simulink model "dqn_C_PQ_HVsMC"  (R2024a)
settings: Solver=FixedStepDiscrete  StartTime=0.0  StopTime=10  FixedStep=Ts_Power  RelTol=1e-3
PreLoadFcn:
  | % HVDCMMCInterconnectionParam
StartFcn:
  | tic
StopFcn:
  | toc
values from neighbouring files (symbols this model uses):
  C_PM = 1.758e-3    (= 0.001758)    [dqnMMCsingle.m]
  Fnom = 50    [dqnMMCsingle.m]
  HRM = 1    [dqnMMCsingle.m]
  Ki_Ireg = 6    [dqnMMCsingle.m]
  Ki_Qreg = 1.0    (= 1)    [dqnMMCsingle.m]
  Kp_Ireg = 0.6    [dqnMMCsingle.m]
  Kp_Qreg = 0.5/3    (= 0.166666666667)    [dqnMMCsingle.m]
  Larm = Larm_pu*(Zb_ac/(2*pi*Fnom))    [dqnMMCsingle.m]
  Larm_pu = 0.15    [dqnMMCsingle.m]
  Lff = Larm_pu/2    (= 0.075)    [dqnMMCsingle.m]
  Limits_Ireg = [ 2.0  -2.0]    [dqnMMCsingle.m]
  Limits_Qreg = [ 0.25, -0.25 ]    [dqnMMCsingle.m]
  Limits_VDCreg = [ 2.0  -2.0]    [dqnMMCsingle.m]
  Lxfo = 0.12    [dqnMMCsingle.m]
  N = 1    [dqnMMCsingle.m]
  Nb_PM = 36    [dqnMMCsingle.m]
  Pnom = 1000e6    (= 1000000000)    [dqnMMCsingle.m]
  R_startup = 400    [dqnMMCsingle.m]
  Rarm = Rarm_pu*Zb_ac    [dqnMMCsingle.m]
  Rff = Rarm_pu/2    (= 0.00075)    [dqnMMCsingle.m]
  Rxfo = 0.003    [dqnMMCsingle.m]
  Slope_Qref = 0.5    [dqnMMCsingle.m]
  Slope_Vdc_ref = Vnom_dc/5    (= 128000)    [dqnMMCsingle.m]
  Tfault = 9999    [dqnMMCsingle.m]
  Ts = Ts_Control    (= 4e-05)    [dqnMMCsingle.m]
  Ts_Control = 40e-6    (= 4e-05)    [dqnMMCsingle.m]
  Ts_dqn = 2e-5    (= 2e-05)    [dqnMMCsingle.m]
  Ts_Power = 20e-6    (= 2e-05)    [dqnMMCsingle.m]
  Vnom_dc = 640e3    (= 640000)    [dqnMMCsingle.m]
  Vnom_prim = 400e3    (= 400000)    [dqnMMCsingle.m]
  Vnom_sec = 333e3    (= 333000)    [dqnMMCsingle.m]
  Ws = 2*pi*50    (= 314.159265359)    [dqnMMCsingle.m]
undefined symbols (not defined in the file or in its folder): DiscIntNeverNeededParam, Discrete, DQN_Lib, gcbh, Int_DQNc_Mat, Mult_DQNc_Mat, Pcc, S, sps, sps_rtmsupport, spsMeanValueVariableFrequencyModel, spsPLL3phModel, SY3
libraries: simulink x18, spsControlledVoltageSourceLib x15, spsVoltageMeasurementLib x9, powerlib_extras x6, spsSecondOrderFilterLib x6, spsCurrentMeasurementLib x6, spsIdealSwitchLib x6, spsMeanLib x4, spsdq0toabcLib x4, spsMeanVariableFrequencyLib x4, spsabctodq0Lib x4, spsThreePhaseSeriesRLCBranchLib x4
(part 3 of 6)

== system dqn_C_PQ_HVsMC/Controllers1/Current Regulator (Ireg)/PI regulator with anti-windup Q ==
  note: Anti-windup mechanism: Method of conditionnal integration
      |
      | The integration is suspended if saturation occurs and the
      | control error is of the same sign as the control signal.
      |
      | [1] L.Rundqwist, "Anti-Reset Windup for PID Controllers," Ph.D. Thesis TRFT-1033,
      | Departement of Automatic Control, Lund Institute of Technology, Lund, Sweeden, 1991.
  Error : Inport  SampleTime=Ts
  Compare To Zero : simulink/Logic and Bit Operations/Compare To Zero  relop=>  OutDataTypeStr=uint8  ZeroCross=off
  Compare To Zero1 : simulink/Logic and Bit Operations/Compare To Zero  relop=<  OutDataTypeStr=uint8  ZeroCross=off
  Constant : Constant  Value=0
  Constant1 : Constant  Value=UpperLimit
  Constant3 : Constant  Value=LowerLimit
  Discrete-Time Integrator : DiscreteIntegrator  IntegratorMethod=Integration: Trapezoidal  InitialCondition=Init  SampleTime=Ts  LimitOutput=on  UpperSaturationLimit=UpperLimit  LowerSaturationLimit=LowerLimit  ShowStatePort=on  ICPrevOutput=DiscIntNeverNeededParam  ICPrevScaledInput=DiscIntNeverNeededParam
  Kp4 : Gain  Gain=Kp  SaturateOnIntegerOverflow=on  SampleTime=Ts  OutDataTypeStr=Inherit: Same as input  ParamDataTypeStr=Inherit: Same as input
  Kp5 : Gain  Gain=Ki  SaturateOnIntegerOverflow=on  SampleTime=Ts  OutDataTypeStr=Inherit: Same as input  ParamDataTypeStr=Inherit: Same as input
  Logical Operator : Logic  AllPortsSameDT=off  OutDataTypeStr=boolean
  Logical Operator1 : Logic  AllPortsSameDT=off  OutDataTypeStr=boolean
  Logical Operator2 : Logic  Operator=OR  AllPortsSameDT=off  OutDataTypeStr=boolean
  Relational Operator : RelationalOperator  OutDataTypeStr=boolean  InputSameDT=off
  Relational Operator1 : RelationalOperator  Operator=<=  OutDataTypeStr=boolean  InputSameDT=off
  Saturation2 : Saturate  UpperLimit=UpperLimit  LowerLimit=LowerLimit  SampleTime=Ts
  Sum1 : Sum  InputSameDT=on  SaturateOnIntegerOverflow=on  SampleTime=Ts  OutDataTypeStr=Inherit: Same as first input
  Sum6 : Sum  InputSameDT=on  SaturateOnIntegerOverflow=on  SampleTime=Ts  OutDataTypeStr=Inherit: Same as first input
  Switch : Switch  Criteria=u2 > Threshold  SaturateOnIntegerOverflow=off  InputSameDT=off
  Zero-Order Hold : ZeroOrderHold  SampleTime=Ts
  Out : Outport  SampleTime=Ts  InitialOutput=0
  wires:
  Kp5/1 -> Switch/3
  Switch/1 -> Discrete-Time Integrator/1
  Saturation2/1 -> Out/1
  Discrete-Time Integrator/1 -> Sum6/2
  Kp4/1 -> Zero-Order Hold/1
  Sum6/1 -> Saturation2/1
  Error/1 -> Kp5/1, Kp4/1, Compare To Zero/1, Compare To Zero1/1
  Compare To Zero1/1 -> Logical Operator1/2  "Error_is_negative"
  Logical Operator1/1 -> Logical Operator2/2
  Logical Operator/1 -> Logical Operator2/1
  Compare To Zero/1 -> Logical Operator/2  "Error_is_positive"
  Constant3/1 -> Relational Operator1/2
  Constant1/1 -> Relational Operator/2
  Relational Operator1/1 -> Logical Operator1/1  "LowerLimit_Is_Reached"
  Relational Operator/1 -> Logical Operator/1  "UpperLimit_is_Reached"
  Logical Operator2/1 -> Switch/2
  Sum1/1 -> Relational Operator/1, Relational Operator1/1
  Discrete-Time Integrator/State -> Sum1/1
  Zero-Order Hold/1 -> Sum6/1, Sum1/2
  Constant/1 -> Switch/1

== system dqn_C_PQ_HVsMC/DQsym/Circulating current suppression2/PI regulator with anti-windup D ==
  note: Anti-windup mechanism: Method of conditionnal integration
      |
      | The integration is suspended if saturation occurs and the
      | control error is of the same sign as the control signal.
      |
      | [1] L.Rundqwist, "Anti-Reset Windup for PID Controllers," Ph.D. Thesis TRFT-1033,
      | Departement of Automatic Control, Lund Institute of Technology, Lund, Sweeden, 1991.
  Error : Inport  SampleTime=Ts
  Compare To Zero : simulink/Logic and Bit Operations/Compare To Zero  relop=>  OutDataTypeStr=uint8  ZeroCross=off
  Compare To Zero1 : simulink/Logic and Bit Operations/Compare To Zero  relop=<  OutDataTypeStr=uint8  ZeroCross=off
  Constant : Constant  Value=0
  Constant1 : Constant  Value=UpperLimit
  Constant3 : Constant  Value=LowerLimit
  Discrete-Time Integrator : DiscreteIntegrator  IntegratorMethod=Integration: Trapezoidal  InitialCondition=Init  SampleTime=Ts  LimitOutput=on  UpperSaturationLimit=UpperLimit  LowerSaturationLimit=LowerLimit  ShowStatePort=on  ICPrevOutput=DiscIntNeverNeededParam  ICPrevScaledInput=DiscIntNeverNeededParam
  Kp4 : Gain  Gain=Kp  SaturateOnIntegerOverflow=on  SampleTime=Ts  OutDataTypeStr=Inherit: Same as input  ParamDataTypeStr=Inherit: Same as input
  Kp5 : Gain  Gain=Ki  SaturateOnIntegerOverflow=on  SampleTime=Ts  OutDataTypeStr=Inherit: Same as input  ParamDataTypeStr=Inherit: Same as input
  Logical Operator : Logic  AllPortsSameDT=off  OutDataTypeStr=boolean
  Logical Operator1 : Logic  AllPortsSameDT=off  OutDataTypeStr=boolean
  Logical Operator2 : Logic  Operator=OR  AllPortsSameDT=off  OutDataTypeStr=boolean
  Relational Operator : RelationalOperator  OutDataTypeStr=boolean  InputSameDT=off
  Relational Operator1 : RelationalOperator  Operator=<=  OutDataTypeStr=boolean  InputSameDT=off
  Saturation2 : Saturate  UpperLimit=UpperLimit  LowerLimit=LowerLimit  SampleTime=Ts
  Sum1 : Sum  InputSameDT=on  SaturateOnIntegerOverflow=on  SampleTime=Ts  OutDataTypeStr=Inherit: Same as first input
  Sum6 : Sum  InputSameDT=on  SaturateOnIntegerOverflow=on  SampleTime=Ts  OutDataTypeStr=Inherit: Same as first input
  Switch : Switch  Criteria=u2 > Threshold  SaturateOnIntegerOverflow=off  InputSameDT=off
  Zero-Order Hold : ZeroOrderHold  SampleTime=Ts
  Out : Outport  SampleTime=Ts  InitialOutput=0
  wires:
  Constant/1 -> Switch/1
  Zero-Order Hold/1 -> Sum1/2, Sum6/1
  Discrete-Time Integrator/State -> Sum1/1
  Sum1/1 -> Relational Operator1/1, Relational Operator/1
  Logical Operator2/1 -> Switch/2
  Relational Operator/1 -> Logical Operator/1  "UpperLimit_is_Reached"
  Relational Operator1/1 -> Logical Operator1/1  "LowerLimit_Is_Reached"
  Constant1/1 -> Relational Operator/2
  Constant3/1 -> Relational Operator1/2
  Compare To Zero/1 -> Logical Operator/2  "Error_is_positive"
  Logical Operator/1 -> Logical Operator2/1
  Logical Operator1/1 -> Logical Operator2/2
  Compare To Zero1/1 -> Logical Operator1/2  "Error_is_negative"
  Error/1 -> Compare To Zero1/1, Compare To Zero/1, Kp4/1, Kp5/1
  Sum6/1 -> Saturation2/1
  Kp4/1 -> Zero-Order Hold/1
  Discrete-Time Integrator/1 -> Sum6/2
  Saturation2/1 -> Out/1
  Switch/1 -> Discrete-Time Integrator/1
  Kp5/1 -> Switch/3

== system dqn_C_PQ_HVsMC/DQsym/Circulating current suppression2/PI regulator with anti-windup D1 ==
  note: Anti-windup mechanism: Method of conditionnal integration
      |
      | The integration is suspended if saturation occurs and the
      | control error is of the same sign as the control signal.
      |
      | [1] L.Rundqwist, "Anti-Reset Windup for PID Controllers," Ph.D. Thesis TRFT-1033,
      | Departement of Automatic Control, Lund Institute of Technology, Lund, Sweeden, 1991.
  Error : Inport  SampleTime=Ts
  Compare To Zero : simulink/Logic and Bit Operations/Compare To Zero  relop=>  OutDataTypeStr=uint8  ZeroCross=off
  Compare To Zero1 : simulink/Logic and Bit Operations/Compare To Zero  relop=<  OutDataTypeStr=uint8  ZeroCross=off
  Constant : Constant  Value=0
  Constant1 : Constant  Value=UpperLimit
  Constant3 : Constant  Value=LowerLimit
  Discrete-Time Integrator : DiscreteIntegrator  IntegratorMethod=Integration: Trapezoidal  InitialCondition=Init  SampleTime=Ts  LimitOutput=on  UpperSaturationLimit=UpperLimit  LowerSaturationLimit=LowerLimit  ShowStatePort=on  ICPrevOutput=DiscIntNeverNeededParam  ICPrevScaledInput=DiscIntNeverNeededParam
  Kp4 : Gain  Gain=Kp  SaturateOnIntegerOverflow=on  SampleTime=Ts  OutDataTypeStr=Inherit: Same as input  ParamDataTypeStr=Inherit: Same as input
  Kp5 : Gain  Gain=Ki  SaturateOnIntegerOverflow=on  SampleTime=Ts  OutDataTypeStr=Inherit: Same as input  ParamDataTypeStr=Inherit: Same as input
  Logical Operator : Logic  AllPortsSameDT=off  OutDataTypeStr=boolean
  Logical Operator1 : Logic  AllPortsSameDT=off  OutDataTypeStr=boolean
  Logical Operator2 : Logic  Operator=OR  AllPortsSameDT=off  OutDataTypeStr=boolean
  Relational Operator : RelationalOperator  OutDataTypeStr=boolean  InputSameDT=off
  Relational Operator1 : RelationalOperator  Operator=<=  OutDataTypeStr=boolean  InputSameDT=off
  Saturation2 : Saturate  UpperLimit=UpperLimit  LowerLimit=LowerLimit  SampleTime=Ts
  Sum1 : Sum  InputSameDT=on  SaturateOnIntegerOverflow=on  SampleTime=Ts  OutDataTypeStr=Inherit: Same as first input
  Sum6 : Sum  InputSameDT=on  SaturateOnIntegerOverflow=on  SampleTime=Ts  OutDataTypeStr=Inherit: Same as first input
  Switch : Switch  Criteria=u2 > Threshold  SaturateOnIntegerOverflow=off  InputSameDT=off
  Zero-Order Hold : ZeroOrderHold  SampleTime=Ts
  Out : Outport  SampleTime=Ts  InitialOutput=0
  wires:
  Kp5/1 -> Switch/3
  Switch/1 -> Discrete-Time Integrator/1
  Saturation2/1 -> Out/1
  Discrete-Time Integrator/1 -> Sum6/2
  Kp4/1 -> Zero-Order Hold/1
  Sum6/1 -> Saturation2/1
  Error/1 -> Kp5/1, Kp4/1, Compare To Zero/1, Compare To Zero1/1
  Compare To Zero1/1 -> Logical Operator1/2  "Error_is_negative"
  Logical Operator1/1 -> Logical Operator2/2
  Logical Operator/1 -> Logical Operator2/1
  Compare To Zero/1 -> Logical Operator/2  "Error_is_positive"
  Constant3/1 -> Relational Operator1/2
  Constant1/1 -> Relational Operator/2
  Relational Operator1/1 -> Logical Operator1/1  "LowerLimit_Is_Reached"
  Relational Operator/1 -> Logical Operator/1  "UpperLimit_is_Reached"
  Logical Operator2/1 -> Switch/2
  Sum1/1 -> Relational Operator/1, Relational Operator1/1
  Discrete-Time Integrator/State -> Sum1/1
  Zero-Order Hold/1 -> Sum6/1, Sum1/2
  Constant/1 -> Switch/1

== system dqn_C_PQ_HVsMC/MMC AVG/Circulating current suppression/PI regulator with anti-windup D ==
  note: Anti-windup mechanism: Method of conditionnal integration
      |
      | The integration is suspended if saturation occurs and the
      | control error is of the same sign as the control signal.
      |
      | [1] L.Rundqwist, "Anti-Reset Windup for PID Controllers," Ph.D. Thesis TRFT-1033,
      | Departement of Automatic Control, Lund Institute of Technology, Lund, Sweeden, 1991.
  Error : Inport  SampleTime=Ts
  Compare To Zero : simulink/Logic and Bit Operations/Compare To Zero  relop=>  OutDataTypeStr=uint8  ZeroCross=off
  Compare To Zero1 : simulink/Logic and Bit Operations/Compare To Zero  relop=<  OutDataTypeStr=uint8  ZeroCross=off
  Constant : Constant  Value=0
  Constant1 : Constant  Value=UpperLimit
  Constant3 : Constant  Value=LowerLimit
  Discrete-Time Integrator : DiscreteIntegrator  IntegratorMethod=Integration: Trapezoidal  InitialCondition=Init  SampleTime=Ts  LimitOutput=on  UpperSaturationLimit=UpperLimit  LowerSaturationLimit=LowerLimit  ShowStatePort=on  ICPrevOutput=DiscIntNeverNeededParam  ICPrevScaledInput=DiscIntNeverNeededParam
  Kp4 : Gain  Gain=Kp  SaturateOnIntegerOverflow=on  SampleTime=Ts  OutDataTypeStr=Inherit: Same as input  ParamDataTypeStr=Inherit: Same as input
  Kp5 : Gain  Gain=Ki  SaturateOnIntegerOverflow=on  SampleTime=Ts  OutDataTypeStr=Inherit: Same as input  ParamDataTypeStr=Inherit: Same as input
  Logical Operator : Logic  AllPortsSameDT=off  OutDataTypeStr=boolean
  Logical Operator1 : Logic  AllPortsSameDT=off  OutDataTypeStr=boolean
  Logical Operator2 : Logic  Operator=OR  AllPortsSameDT=off  OutDataTypeStr=boolean
  Relational Operator : RelationalOperator  OutDataTypeStr=boolean  InputSameDT=off
  Relational Operator1 : RelationalOperator  Operator=<=  OutDataTypeStr=boolean  InputSameDT=off
  Saturation2 : Saturate  UpperLimit=UpperLimit  LowerLimit=LowerLimit  SampleTime=Ts
  Sum1 : Sum  InputSameDT=on  SaturateOnIntegerOverflow=on  SampleTime=Ts  OutDataTypeStr=Inherit: Same as first input
  Sum6 : Sum  InputSameDT=on  SaturateOnIntegerOverflow=on  SampleTime=Ts  OutDataTypeStr=Inherit: Same as first input
  Switch : Switch  Criteria=u2 > Threshold  SaturateOnIntegerOverflow=off  InputSameDT=off
  Zero-Order Hold : ZeroOrderHold  SampleTime=Ts
  Out : Outport  SampleTime=Ts  InitialOutput=0
  wires:
  Constant/1 -> Switch/1
  Zero-Order Hold/1 -> Sum1/2, Sum6/1
  Discrete-Time Integrator/State -> Sum1/1
  Sum1/1 -> Relational Operator1/1, Relational Operator/1
  Logical Operator2/1 -> Switch/2
  Relational Operator/1 -> Logical Operator/1  "UpperLimit_is_Reached"
  Relational Operator1/1 -> Logical Operator1/1  "LowerLimit_Is_Reached"
  Constant1/1 -> Relational Operator/2
  Constant3/1 -> Relational Operator1/2
  Compare To Zero/1 -> Logical Operator/2  "Error_is_positive"
  Logical Operator/1 -> Logical Operator2/1
  Logical Operator1/1 -> Logical Operator2/2
  Compare To Zero1/1 -> Logical Operator1/2  "Error_is_negative"
  Error/1 -> Compare To Zero1/1, Compare To Zero/1, Kp4/1, Kp5/1
  Sum6/1 -> Saturation2/1
  Kp4/1 -> Zero-Order Hold/1
  Discrete-Time Integrator/1 -> Sum6/2
  Saturation2/1 -> Out/1
  Switch/1 -> Discrete-Time Integrator/1
  Kp5/1 -> Switch/3

== system dqn_C_PQ_HVsMC/MMC AVG/Circulating current suppression/PI regulator with anti-windup D1 ==
  note: Anti-windup mechanism: Method of conditionnal integration
      |
      | The integration is suspended if saturation occurs and the
      | control error is of the same sign as the control signal.
      |
      | [1] L.Rundqwist, "Anti-Reset Windup for PID Controllers," Ph.D. Thesis TRFT-1033,
      | Departement of Automatic Control, Lund Institute of Technology, Lund, Sweeden, 1991.
  Error : Inport  SampleTime=Ts
  Compare To Zero : simulink/Logic and Bit Operations/Compare To Zero  relop=>  OutDataTypeStr=uint8  ZeroCross=off
  Compare To Zero1 : simulink/Logic and Bit Operations/Compare To Zero  relop=<  OutDataTypeStr=uint8  ZeroCross=off
  Constant : Constant  Value=0
  Constant1 : Constant  Value=UpperLimit
  Constant3 : Constant  Value=LowerLimit
  Discrete-Time Integrator : DiscreteIntegrator  IntegratorMethod=Integration: Trapezoidal  InitialCondition=Init  SampleTime=Ts  LimitOutput=on  UpperSaturationLimit=UpperLimit  LowerSaturationLimit=LowerLimit  ShowStatePort=on  ICPrevOutput=DiscIntNeverNeededParam  ICPrevScaledInput=DiscIntNeverNeededParam
  Kp4 : Gain  Gain=Kp  SaturateOnIntegerOverflow=on  SampleTime=Ts  OutDataTypeStr=Inherit: Same as input  ParamDataTypeStr=Inherit: Same as input
  Kp5 : Gain  Gain=Ki  SaturateOnIntegerOverflow=on  SampleTime=Ts  OutDataTypeStr=Inherit: Same as input  ParamDataTypeStr=Inherit: Same as input
  Logical Operator : Logic  AllPortsSameDT=off  OutDataTypeStr=boolean
  Logical Operator1 : Logic  AllPortsSameDT=off  OutDataTypeStr=boolean
  Logical Operator2 : Logic  Operator=OR  AllPortsSameDT=off  OutDataTypeStr=boolean
  Relational Operator : RelationalOperator  OutDataTypeStr=boolean  InputSameDT=off
  Relational Operator1 : RelationalOperator  Operator=<=  OutDataTypeStr=boolean  InputSameDT=off
  Saturation2 : Saturate  UpperLimit=UpperLimit  LowerLimit=LowerLimit  SampleTime=Ts
  Sum1 : Sum  InputSameDT=on  SaturateOnIntegerOverflow=on  SampleTime=Ts  OutDataTypeStr=Inherit: Same as first input
  Sum6 : Sum  InputSameDT=on  SaturateOnIntegerOverflow=on  SampleTime=Ts  OutDataTypeStr=Inherit: Same as first input
  Switch : Switch  Criteria=u2 > Threshold  SaturateOnIntegerOverflow=off  InputSameDT=off
  Zero-Order Hold : ZeroOrderHold  SampleTime=Ts
  Out : Outport  SampleTime=Ts  InitialOutput=0
  wires:
  Kp5/1 -> Switch/3
  Switch/1 -> Discrete-Time Integrator/1
  Saturation2/1 -> Out/1
  Discrete-Time Integrator/1 -> Sum6/2
  Kp4/1 -> Zero-Order Hold/1
  Sum6/1 -> Saturation2/1
  Error/1 -> Kp5/1, Kp4/1, Compare To Zero/1, Compare To Zero1/1
  Compare To Zero1/1 -> Logical Operator1/2  "Error_is_negative"
  Logical Operator1/1 -> Logical Operator2/2
  Logical Operator/1 -> Logical Operator2/1
  Compare To Zero/1 -> Logical Operator/2  "Error_is_positive"
  Constant3/1 -> Relational Operator1/2
  Constant1/1 -> Relational Operator/2
  Relational Operator1/1 -> Logical Operator1/1  "LowerLimit_Is_Reached"
  Relational Operator/1 -> Logical Operator/1  "UpperLimit_is_Reached"
  Logical Operator2/1 -> Switch/2
  Sum1/1 -> Relational Operator/1, Relational Operator1/1
  Discrete-Time Integrator/State -> Sum1/1
  Zero-Order Hold/1 -> Sum6/1, Sum1/2
  Constant/1 -> Switch/1

== system dqn_C_PQ_HVsMC/MMC AVG/Subsystem/Subsystem ==
  g : Inport
  cb1 : spsIdealSwitchLib/Ideal Switch  Ron=0.001  Lon=0  IC=0  Rs=1e6  Cs=inf  Measurements=off
  cb2 : spsIdealSwitchLib/Ideal Switch  Ron=0.001  Lon=0  IC=0  Rs=1e6  Cs=inf  Measurements=off
  cb3 : spsIdealSwitchLib/Ideal Switch  Ron=0.001  Lon=0  IC=0  Rs=1e6  Cs=inf  Measurements=off
  1 : PMIOPort  Side=Left
  2 : PMIOPort  Port=2  Side=Left
  3 : PMIOPort  Port=3  Side=Left
  4 : PMIOPort  Port=4  Side=Right
  5 : PMIOPort  Port=5  Side=Right
  6 : PMIOPort  Port=6  Side=Right
  wires:
  g/1 -> cb3/1, cb2/1, cb1/1
  connections:
  cb3/RConn1 -- 6/RConn1
  cb3/LConn1 -- 3/RConn1
  cb2/RConn1 -- 5/RConn1
  cb1/LConn1 -- 1/RConn1
  cb1/RConn1 -- 4/RConn1
  cb2/LConn1 -- 2/RConn1

== system dqn_C_PQ_HVsMC/MMC AVG/Subsystem/Subsystem1 ==
  g : Inport
  cb4 : spsIdealSwitchLib/Ideal Switch  Ron=0.001  Lon=0  IC=0  Rs=1e6  Cs=inf  Measurements=off
  cb5 : spsIdealSwitchLib/Ideal Switch  Ron=0.001  Lon=0  IC=0  Rs=1e6  Cs=inf  Measurements=off
  cb6 : spsIdealSwitchLib/Ideal Switch  Ron=0.001  Lon=0  IC=0  Rs=1e6  Cs=inf  Measurements=off
  1 : PMIOPort  Side=Left
  2 : PMIOPort  Port=2  Side=Left
  3 : PMIOPort  Port=3  Side=Left
  4 : PMIOPort  Port=4  Side=Right
  5 : PMIOPort  Port=5  Side=Right
  6 : PMIOPort  Port=6  Side=Right
  wires:
  g/1 -> cb6/1, cb5/1, cb4/1
  connections:
  cb6/RConn1 -- 6/RConn1
  cb6/LConn1 -- 3/RConn1
  cb5/RConn1 -- 5/RConn1
  cb4/LConn1 -- 1/RConn1
  cb4/RConn1 -- 4/RConn1
  cb5/LConn1 -- 2/RConn1

== system dqn_C_PQ_HVsMC/Control _DQn/PLL, Measurements and Transformation1/PLL (3ph)/Model ==
  note: vq
  Vdq : Inport
  Automatic Gain Control : Subsystem  TreatAsAtomicUnit=on
  Constant1 : Constant  Value=sps.AGC  SampleTime=Ts
  Constant4 : Constant  Value=2*pi  SampleTime=Ts
  Discrete : Subsystem  DialogController=POWERSYS.PowerSysDialog  VariantControl=PID_Discrete  mask(Discrete PID Controller){Kp=sps.Kp, Ki=sps.Ki, Kd=sps.Kd, TcD=sps.TcD, Par_Limits=[inf 0], Init=2*pi*sps.Finit, Ts=Ts}
      mask prompts: Kp "Proportional gain (Kp):"; Ki "Integral gain (Ki):"; Kd "Derivative gain (Kd):"; TcD "Time constant for derivative filter (s):"; Par_Limits "Output limits: [ Upper   Lower ]"; Init "Output initial value:"; Ts "Sample time:"
      mask help: This block implements a discrete PID controller.
      mask Display: disp('PID');
  Discrete-Time Integrator : DiscreteIntegrator  ExternalReset=rising  InitialConditionSource=external  InitialCondition=sps.Phase_Init*pi/180  SampleTime=Ts  ShowStatePort=on  ICPrevOutput=DiscIntNeverNeededParam  ICPrevScaledInput=DiscIntNeverNeededParam
  Divide : Product
  Gain10 : Gain  Gain=1/2/pi  SaturateOnIntegerOverflow=on  OutDataTypeStr=Inherit: Same as input  ParamDataTypeStr=Inherit: Same as input
  Initial : InitialCondition  Value=sps.Phase_Init*pi/180
  Rate Limiter : RateLimiter  RisingSlewLimit=sps.MaxRateChangeFreq  FallingSlewLimit=-sps.MaxRateChangeFreq  SampleTimeMode=inherited  InitialCondition=sps.Finit
  Relational Operator : RelationalOperator  Operator=>  OutDataTypeStr=boolean  InputSameDT=off
  Second-Order Filter : spsSecondOrderFilterLib/Second-Order Filter  FilterType=Lowpass  Fo=sps.FilterCutOffFreq  Zeta=0.707  Ts=Ts  Initialize=on  Vac_Init=[0 0 sps.Finit]  Vdc_Init=sps.Finit  PlotResponse=off  FreqRange=[1 500 1]
      settings: LibrarySourceBlock=|
      | sps_lib/Control/Filters/Second-Order
      | Filter
  Selector : Selector  Commented=on  InputPortWidth=3  IndexOptions=Index vector (dialog)  Indices=2  OutputSizes=1
  Selector1 : Selector  InputPortWidth=2  IndexOptions=Index vector (dialog)  Indices=2  OutputSizes=1
  Subtract : Sum  Inputs=+-
  Unit Delay : UnitDelay  InitialCondition=sps.Finit  SampleTime=Ts  HasFrameUpgradeWarning=on
  Variable Frequency Mean value : Subsystem  AncestorBlock=|  DialogController=POWERSYS.PowerSysDialog  LoadFcn=sps_rtmsupport('LoadFcn', gcbh);  StartFcn=sps_rtmsupport('StartFcn', gcbh);  StopFcn=sps_rtmsupport('StopFcn', gcbh);  mask(Mean (Variable Frequency)){Finit=sps.Finit, Fmin=sps.Fmin, Vinit=0, Ts=Ts}
      | sps_lib/Sensors and Measurements/Mean
      | (Variable Frequency)
      mask prompts: Finit "Initial frequency (Hz):"; Fmin "Minimum frequency (Hz):"; Vinit "Initial input (DC component):"; Ts "Sample time:"
      mask help:
      | Compute the mean value of input 2 over a running window of one cycle of frequency signal given by input 1.
      |
      | For the first cycle of initial frequency, the output is held to the value specified in the Initial input (DC component) parameter.
      |
      | The Minimum frequency parameter is used to determine the buffer size of the Variable Time Delay block used under the mask of the block.
      mask init:
      | block=gcb;
      | [WantBlockChoice,Ts,sps] = powericon('MeanVariableFrequencyInit',block,Finit,Fmin,Vinit,Ts);
      | powericon('SetInternalModels','set',block,WantBlockChoice);
      settings: CopyFcn=sps_rtmsupport('CopyFcn', gcbh);  DeleteFcn=sps_rtmsupport('DeleteFcn', gcbh);  UndoDeleteFcn=sps_rtmsupport('UndoDeleteFcn', gcbh);  ModelCloseFcn=sps_rtmsupport('ModelCloseFcn', gcbh);  PreSaveFcn=sps_rtmsupport('PreSaveFcn', gcbh);  PostSaveFcn=sps_rtmsupport('PostSaveFcn', gcbh);  NameChangeFcn=sps_rtmsupport('NameChangeFcn', gcbh);  PreCopyFcn=sps_rtmsupport('PreCopyFcn', gcbh);  OpenFcn=sps_rtmsupport('OpenFcn', gcbh, []);  CloseFcn=sps_rtmsupport('CloseFcn', gcbh);  PreDeleteFcn=sps_rtmsupport('PreDeleteFcn', gcbh);
      settings: LibrarySourceBlock=|
      | sps_lib/Sensors and Measurements/Mean
      | (Variable Frequency)
      mask Help: helpview(psbhelp);
      mask Display:
      | port_label('input',1,'Freq')
      | port_label('input',2,'In')
      | plot(0,0, 1,1)
      | plot([0.8 1], [0.75 0.75])
      | plot([0.85 .95], [0.35 0.65],[0.85 .95], [0.65 0.35])
  abc to dq0 : spsabctodq0Lib/abc to dq0  Commented=on  Alignment=90 degrees behind phase A axis
  Freq : Outport  VectorParamsAs1DForOutWhenUnconnected=off
  wt : Outport  Port=2  VectorParamsAs1DForOutWhenUnconnected=off
  wires:
  Rate Limiter/1 -> Second-Order Filter/1
  Gain10/1 -> Rate Limiter/1
  Vdq/1 -> Automatic Gain Control/2(Vdq), Selector1/1
  Second-Order Filter/1 -> Unit Delay/1
  Unit Delay/1 -> Automatic Gain Control/1(Freq), Variable Frequency Mean value/1(Freq), Freq/1
  Discrete-Time Integrator/1 -> wt/1
  Constant4/1 -> Subtract/2, Relational Operator/2
  abc to dq0/1 -> Selector/1
  Discrete/1(Out) -> Gain10/1, Discrete-Time Integrator/1  "W"
  Variable Frequency Mean value/1(Mean) -> Divide/1
  Automatic Gain Control/1(Gain) -> Divide/2
  Divide/1 -> Discrete/1(Err)
  Constant1/1 -> Automatic Gain Control/Enable
  Relational Operator/1 -> Discrete-Time Integrator/2
  Discrete-Time Integrator/State -> Subtract/1, Relational Operator/1
  Subtract/1 -> Initial/1
  Initial/1 -> Discrete-Time Integrator/3
  Selector1/1 -> Variable Frequency Mean value/2(vq)

== system dqn_C_PQ_HVsMC/Control _DQn/PLL, Measurements and Transformation1/PLL (3ph)2/Model ==
  note: vq
  Vdq : Inport
  Automatic Gain Control : Subsystem  TreatAsAtomicUnit=on
  Constant1 : Constant  Value=sps.AGC  SampleTime=Ts
  Constant4 : Constant  Value=2*pi  SampleTime=Ts
  Discrete : Subsystem  DialogController=POWERSYS.PowerSysDialog  VariantControl=PID_Discrete  mask(Discrete PID Controller){Kp=sps.Kp, Ki=sps.Ki, Kd=sps.Kd, TcD=sps.TcD, Par_Limits=[inf 0], Init=2*pi*sps.Finit, Ts=Ts}
      mask prompts: Kp "Proportional gain (Kp):"; Ki "Integral gain (Ki):"; Kd "Derivative gain (Kd):"; TcD "Time constant for derivative filter (s):"; Par_Limits "Output limits: [ Upper   Lower ]"; Init "Output initial value:"; Ts "Sample time:"
      mask help: This block implements a discrete PID controller.
      mask Display: disp('PID');
  Discrete-Time Integrator : DiscreteIntegrator  ExternalReset=rising  InitialConditionSource=external  InitialCondition=sps.Phase_Init*pi/180  SampleTime=Ts  ShowStatePort=on  ICPrevOutput=DiscIntNeverNeededParam  ICPrevScaledInput=DiscIntNeverNeededParam
  Divide : Product
  Gain10 : Gain  Gain=1/2/pi  SaturateOnIntegerOverflow=on  OutDataTypeStr=Inherit: Same as input  ParamDataTypeStr=Inherit: Same as input
  Initial : InitialCondition  Value=sps.Phase_Init*pi/180
  MATLAB Function : MATLAB Function  TreatAsAtomicUnit=on
  Mux : Mux  Inputs=2
  Rate Limiter : RateLimiter  RisingSlewLimit=sps.MaxRateChangeFreq  FallingSlewLimit=-sps.MaxRateChangeFreq  SampleTimeMode=inherited  InitialCondition=sps.Finit
  Rate Transition3 : RateTransition  OutPortSampleTime=Ts_Control
  Relational Operator : RelationalOperator  Operator=>  OutDataTypeStr=boolean  InputSameDT=off
  Second-Order Filter : spsSecondOrderFilterLib/Second-Order Filter  FilterType=Lowpass  Fo=sps.FilterCutOffFreq  Zeta=0.707  Ts=Ts  Initialize=on  Vac_Init=[0 0 sps.Finit]  Vdc_Init=sps.Finit  PlotResponse=off  FreqRange=[1 500 1]
      settings: LibrarySourceBlock=|
      | sps_lib/Control/Filters/Second-Order
      | Filter
  Selector1 : Selector  InputPortWidth=2  IndexOptions=Index vector (dialog)  Indices=2  OutputSizes=1
  Subtract : Sum  Inputs=+-
  Sum : Sum  Inputs=|+-
  Unit Delay : UnitDelay  InitialCondition=sps.Finit  SampleTime=Ts  HasFrameUpgradeWarning=on
  Variable Frequency Mean value : Subsystem  AncestorBlock=|  DialogController=POWERSYS.PowerSysDialog  LoadFcn=sps_rtmsupport('LoadFcn', gcbh);  StartFcn=sps_rtmsupport('StartFcn', gcbh);  StopFcn=sps_rtmsupport('StopFcn', gcbh);  mask(Mean (Variable Frequency)){Finit=sps.Finit, Fmin=sps.Fmin, Vinit=0, Ts=Ts}
      | sps_lib/Sensors and Measurements/Mean
      | (Variable Frequency)
      mask prompts: Finit "Initial frequency (Hz):"; Fmin "Minimum frequency (Hz):"; Vinit "Initial input (DC component):"; Ts "Sample time:"
      mask help:
      | Compute the mean value of input 2 over a running window of one cycle of frequency signal given by input 1.
      |
      | For the first cycle of initial frequency, the output is held to the value specified in the Initial input (DC component) parameter.
      |
      | The Minimum frequency parameter is used to determine the buffer size of the Variable Time Delay block used under the mask of the block.
      mask init:
      | block=gcb;
      | [WantBlockChoice,Ts,sps] = powericon('MeanVariableFrequencyInit',block,Finit,Fmin,Vinit,Ts);
      | powericon('SetInternalModels','set',block,WantBlockChoice);
      settings: CopyFcn=sps_rtmsupport('CopyFcn', gcbh);  DeleteFcn=sps_rtmsupport('DeleteFcn', gcbh);  UndoDeleteFcn=sps_rtmsupport('UndoDeleteFcn', gcbh);  ModelCloseFcn=sps_rtmsupport('ModelCloseFcn', gcbh);  PreSaveFcn=sps_rtmsupport('PreSaveFcn', gcbh);  PostSaveFcn=sps_rtmsupport('PostSaveFcn', gcbh);  NameChangeFcn=sps_rtmsupport('NameChangeFcn', gcbh);  PreCopyFcn=sps_rtmsupport('PreCopyFcn', gcbh);  OpenFcn=sps_rtmsupport('OpenFcn', gcbh, []);  CloseFcn=sps_rtmsupport('CloseFcn', gcbh);  PreDeleteFcn=sps_rtmsupport('PreDeleteFcn', gcbh);
      settings: LibrarySourceBlock=|
      | sps_lib/Sensors and Measurements/Mean
      | (Variable Frequency)
      mask Help: helpview(psbhelp);
      mask Display:
      | port_label('input',1,'Freq')
      | port_label('input',2,'In')
      | plot(0,0, 1,1)
      | plot([0.8 1], [0.75 0.75])
      | plot([0.85 .95], [0.35 0.65],[0.85 .95], [0.65 0.35])
  Freq : Outport  VectorParamsAs1DForOutWhenUnconnected=off
  wt : Outport  Port=2  VectorParamsAs1DForOutWhenUnconnected=off
  wires:
  Rate Limiter/1 -> Second-Order Filter/1
  Gain10/1 -> Rate Limiter/1
  Second-Order Filter/1 -> Unit Delay/1
  Unit Delay/1 -> Automatic Gain Control/1(Freq), Variable Frequency Mean value/1(Freq), Freq/1
  Constant4/1 -> Subtract/2, Relational Operator/2
  Discrete/1(Out) -> Gain10/1, Discrete-Time Integrator/1  "W"
  Variable Frequency Mean value/1(Mean) -> Divide/1
  Automatic Gain Control/1(Gain) -> Divide/2
  Divide/1 -> Discrete/1(Err)
  Constant1/1 -> Automatic Gain Control/Enable
  Relational Operator/1 -> Discrete-Time Integrator/2
  Discrete-Time Integrator/State -> Subtract/1, Relational Operator/1
  Subtract/1 -> Initial/1
  Initial/1 -> Discrete-Time Integrator/3
  Selector1/1 -> Variable Frequency Mean value/2(vq)
  Sum/1 -> MATLAB Function/2(wt)
  Discrete-Time Integrator/1 -> Sum/1, wt/1
  MATLAB Function/1(d) -> Mux/1
  MATLAB Function/2(q) -> Mux/2
  Mux/1 -> Automatic Gain Control/2(Vdq), Selector1/1
  Vdq/1 -> MATLAB Function/1(DQ)
  [wt0] -> Rate Transition3/1
  Rate Transition3/1 -> Sum/2

== system dqn_C_PQ_HVsMC/Control _DQn/PLL, Measurements and Transformation1/PLL (3ph)/Model/Automatic Gain Control ==
  Freq : Inport
  Vdq : Inport  Port=2
  Enable : EnablePort  PropagateVarSize=During execution
  Math Function : Math  Operator=reciprocal  SignedPower=on
  Positive-Sequence (PLL-Driven) : Subsystem  AncestorBlock=|  DialogController=POWERSYS.PowerSysDialog  LoadFcn=sps_rtmsupport('LoadFcn', gcbh);  StartFcn=sps_rtmsupport('StartFcn', gcbh);  StopFcn=sps_rtmsupport('StopFcn', gcbh);  mask(Positive-Sequence (PLL-Driven)){Finit=sps.Finit, Fmin=sps.Fmin, InInit=[1 0], Ts=Ts}
      | sps_lib/Sensors and Measurements/Positive-Sequence
      | (PLL-Driven)
      mask prompts: Finit "Initial frequency (Hz):"; Fmin "Minimum frequency (Hz):"; InInit "Initial input (positive component)  [ Mag, Phase-relative-to-PLL (degrees) ]:"; Ts "Sample time:"
      mask help:
      | Compute the positive-sequence component of the input 3 signal over a running window of one cycle of fundamental frequency given by input 1. The signal can be a set of three balanced or unbalanced signals which may contain harmonics.
      | The reference frame required for the computation is given by the input 2.
      |
      | The two outputs return respectively the magnitude (same units as the input 3 signal) and phase (in degrees relative to the PLL phase) of the positive-sequence component of the abc input at the fundamental frequency.
      |
      | For the first cycle of simulation, the outputs are held constant to the values specified by the Initial input parameter. The Minimum frequency parameter is used to determine the buffer size of the Variable Transport Delay block used in the model.
      mask init:
      | [WantBlockChoice,Ts,sps] = powericon('PositiveSequencePLLDrivenInit',gcb,Finit,Fmin,InInit,Ts);
      settings: CopyFcn=sps_rtmsupport('CopyFcn', gcbh);  DeleteFcn=sps_rtmsupport('DeleteFcn', gcbh);  UndoDeleteFcn=sps_rtmsupport('UndoDeleteFcn', gcbh);  ModelCloseFcn=sps_rtmsupport('ModelCloseFcn', gcbh);  PreSaveFcn=sps_rtmsupport('PreSaveFcn', gcbh);  PostSaveFcn=sps_rtmsupport('PostSaveFcn', gcbh);  NameChangeFcn=sps_rtmsupport('NameChangeFcn', gcbh);  PreCopyFcn=sps_rtmsupport('PreCopyFcn', gcbh);  OpenFcn=sps_rtmsupport('OpenFcn', gcbh, []);  CloseFcn=sps_rtmsupport('CloseFcn', gcbh);  PreDeleteFcn=sps_rtmsupport('PreDeleteFcn', gcbh);
      settings: LibrarySourceBlock=|
      | sps_lib/Sensors and Measurements/Positive-Sequence
      | (PLL-Driven)
      mask Help: helpview(psbhelp);
      mask Display:
      | port_label('input',1,'Freq')
      | port_label('input',2,'wt')
      | port_label('input',3,'abc')
      | port_label('output',1,'|u|')
      | port_label('output',2,'\angleu', 'texmode', 'on')
  Saturation : Saturate  UpperLimit=inf  LowerLimit=eps
  Terminator1 : Terminator
  Gain : Outport  InitialOutput=[1]  VectorParamsAs1DForOutWhenUnconnected=off
  wires:
  Positive-Sequence (PLL-Driven)/1(Mag) -> Saturation/1
  Positive-Sequence (PLL-Driven)/2(Phase) -> Terminator1/1
  Math Function/1 -> Gain/1
  Vdq/1 -> Positive-Sequence (PLL-Driven)/2(dq)
  Freq/1 -> Positive-Sequence (PLL-Driven)/1(Freq)
  Saturation/1 -> Math Function/1

== system dqn_C_PQ_HVsMC/Control _DQn/PLL, Measurements and Transformation1/PLL (3ph)/Model/Discrete ==
  Err : Inport  SampleTime=Ts
  "Discrete Derivative " : DiscreteTransferFcn  Numerator="[ 1  -1 ]*Kd"  Denominator="[ TcD  Ts-TcD ]"  SampleTime=Ts
  Discrete-Time Integrator : DiscreteIntegrator  gainval=Ki  InitialCondition=Init  SampleTime=Ts  LimitOutput=on  UpperSaturationLimit=Par_Limits(1)  LowerSaturationLimit=Par_Limits(2)  ICPrevOutput=DiscIntNeverNeededParam  ICPrevScaledInput=DiscIntNeverNeededParam
  Kp4 : Gain  Gain=Kp  SaturateOnIntegerOverflow=on  SampleTime=Ts  OutDataTypeStr=Inherit: Same as input  ParamDataTypeStr=Inherit: Same as input
  Saturation1 : Saturate  UpperLimit=Par_Limits(1)  LowerLimit=Par_Limits(2)  SampleTime=Ts
  Sum6 : Sum  Inputs=+++  InputSameDT=on  SaturateOnIntegerOverflow=on  SampleTime=Ts  OutDataTypeStr=Inherit: Same as first input
  Out : Outport  SampleTime=Ts  InitialOutput=0  VectorParamsAs1DForOutWhenUnconnected=off
  wires:
  "Discrete Derivative "/1 -> Sum6/3
  Discrete-Time Integrator/1 -> Sum6/2
  Kp4/1 -> Sum6/1
  Sum6/1 -> Saturation1/1
  Err/1 -> "Discrete Derivative "/1, Kp4/1, Discrete-Time Integrator/1
  Saturation1/1 -> Out/1

== system dqn_C_PQ_HVsMC/Control _DQn/PLL, Measurements and Transformation1/PLL (3ph)/Model/Variable Frequency Mean value ==
  Freq : Inport  PortDimensions=1  SampleTime=Ts
  vq : Inport  Port=2  SampleTime=Ts
  Model : Subsystem  AncestorBlock=spsMeanValueVariableFrequencyModel/Discrete
  Mean : Outport  SampleTime=Ts  VectorParamsAs1DForOutWhenUnconnected=off
  wires:
  Model/1(Mean) -> Mean/1
  vq/1 -> Model/2(vq)
  Freq/1 -> Model/1(Freq)

== system dqn_C_PQ_HVsMC/Control _DQn/PLL, Measurements and Transformation1/PLL (3ph)2/Model/Automatic Gain Control ==
  Freq : Inport
  Vdq : Inport  Port=2
  Enable : EnablePort  PropagateVarSize=During execution
  Math Function : Math  Operator=reciprocal  SignedPower=on
  Positive-Sequence (PLL-Driven) : Subsystem  AncestorBlock=|  DialogController=POWERSYS.PowerSysDialog  LoadFcn=sps_rtmsupport('LoadFcn', gcbh);  StartFcn=sps_rtmsupport('StartFcn', gcbh);  StopFcn=sps_rtmsupport('StopFcn', gcbh);  mask(Positive-Sequence (PLL-Driven)){Finit=sps.Finit, Fmin=sps.Fmin, InInit=[1 0], Ts=Ts}
      | sps_lib/Sensors and Measurements/Positive-Sequence
      | (PLL-Driven)
      mask prompts: Finit "Initial frequency (Hz):"; Fmin "Minimum frequency (Hz):"; InInit "Initial input (positive component)  [ Mag, Phase-relative-to-PLL (degrees) ]:"; Ts "Sample time:"
      mask help:
      | Compute the positive-sequence component of the input 3 signal over a running window of one cycle of fundamental frequency given by input 1. The signal can be a set of three balanced or unbalanced signals which may contain harmonics.
      | The reference frame required for the computation is given by the input 2.
      |
      | The two outputs return respectively the magnitude (same units as the input 3 signal) and phase (in degrees relative to the PLL phase) of the positive-sequence component of the abc input at the fundamental frequency.
      |
      | For the first cycle of simulation, the outputs are held constant to the values specified by the Initial input parameter. The Minimum frequency parameter is used to determine the buffer size of the Variable Transport Delay block used in the model.
      mask init:
      | [WantBlockChoice,Ts,sps] = powericon('PositiveSequencePLLDrivenInit',gcb,Finit,Fmin,InInit,Ts);
      settings: CopyFcn=sps_rtmsupport('CopyFcn', gcbh);  DeleteFcn=sps_rtmsupport('DeleteFcn', gcbh);  UndoDeleteFcn=sps_rtmsupport('UndoDeleteFcn', gcbh);  ModelCloseFcn=sps_rtmsupport('ModelCloseFcn', gcbh);  PreSaveFcn=sps_rtmsupport('PreSaveFcn', gcbh);  PostSaveFcn=sps_rtmsupport('PostSaveFcn', gcbh);  NameChangeFcn=sps_rtmsupport('NameChangeFcn', gcbh);  PreCopyFcn=sps_rtmsupport('PreCopyFcn', gcbh);  OpenFcn=sps_rtmsupport('OpenFcn', gcbh, []);  CloseFcn=sps_rtmsupport('CloseFcn', gcbh);  PreDeleteFcn=sps_rtmsupport('PreDeleteFcn', gcbh);
      settings: LibrarySourceBlock=|
      | sps_lib/Sensors and Measurements/Positive-Sequence
      | (PLL-Driven)
      mask Help: helpview(psbhelp);
      mask Display:
      | port_label('input',1,'Freq')
      | port_label('input',2,'wt')
      | port_label('input',3,'abc')
      | port_label('output',1,'|u|')
      | port_label('output',2,'\angleu', 'texmode', 'on')
  Saturation : Saturate  UpperLimit=inf  LowerLimit=eps
  Terminator1 : Terminator
  Gain : Outport  InitialOutput=[1]  VectorParamsAs1DForOutWhenUnconnected=off
  wires:
  Positive-Sequence (PLL-Driven)/1(Mag) -> Saturation/1
  Positive-Sequence (PLL-Driven)/2(Phase) -> Terminator1/1
  Math Function/1 -> Gain/1
  Vdq/1 -> Positive-Sequence (PLL-Driven)/2(dq)
  Freq/1 -> Positive-Sequence (PLL-Driven)/1(Freq)
  Saturation/1 -> Math Function/1

== system dqn_C_PQ_HVsMC/Control _DQn/PLL, Measurements and Transformation1/PLL (3ph)2/Model/Discrete ==
  Err : Inport  SampleTime=Ts
  "Discrete Derivative " : DiscreteTransferFcn  Numerator="[ 1  -1 ]*Kd"  Denominator="[ TcD  Ts-TcD ]"  SampleTime=Ts
  Discrete-Time Integrator : DiscreteIntegrator  gainval=Ki  InitialCondition=Init  SampleTime=Ts  LimitOutput=on  UpperSaturationLimit=Par_Limits(1)  LowerSaturationLimit=Par_Limits(2)  ICPrevOutput=DiscIntNeverNeededParam  ICPrevScaledInput=DiscIntNeverNeededParam
  Kp4 : Gain  Gain=Kp  SaturateOnIntegerOverflow=on  SampleTime=Ts  OutDataTypeStr=Inherit: Same as input  ParamDataTypeStr=Inherit: Same as input
  Saturation1 : Saturate  UpperLimit=Par_Limits(1)  LowerLimit=Par_Limits(2)  SampleTime=Ts
  Sum6 : Sum  Inputs=+++  InputSameDT=on  SaturateOnIntegerOverflow=on  SampleTime=Ts  OutDataTypeStr=Inherit: Same as first input
  Out : Outport  SampleTime=Ts  InitialOutput=0  VectorParamsAs1DForOutWhenUnconnected=off
  wires:
  "Discrete Derivative "/1 -> Sum6/3
  Discrete-Time Integrator/1 -> Sum6/2
  Kp4/1 -> Sum6/1
  Sum6/1 -> Saturation1/1
  Err/1 -> "Discrete Derivative "/1, Kp4/1, Discrete-Time Integrator/1
  Saturation1/1 -> Out/1

== system dqn_C_PQ_HVsMC/Control _DQn/PLL, Measurements and Transformation1/PLL (3ph)2/Model/Variable Frequency Mean value ==
  Freq : Inport  PortDimensions=1  SampleTime=Ts
  vq : Inport  Port=2  SampleTime=Ts
  Model : Subsystem  AncestorBlock=spsMeanValueVariableFrequencyModel/Discrete
  Mean : Outport  SampleTime=Ts  VectorParamsAs1DForOutWhenUnconnected=off
  wires:
  Model/1(Mean) -> Mean/1
  vq/1 -> Model/2(vq)
  Freq/1 -> Model/1(Freq)

== system dqn_C_PQ_HVsMC/Control _DQn/PLL, Measurements and Transformation1/PLL (3ph)/Model/Automatic Gain Control/Positive-Sequence (PLL-Driven) ==
  Freq : Inport  SampleTime=Ts
  dq : Inport  Port=2  SampleTime=Ts
  Complex to Magnitude-Angle : ComplexToMagnitudeAngle
  Mean (Variable Frequency)1 : spsMeanVariableFrequencyLib/Mean (Variable Frequency)  Finit=sps.Finit  Fmin=sps.Fmin  Vinit=sps.Real_Init  Ts=Ts
      settings: LibrarySourceBlock=|
      | sps_lib/Sensors and Measurements/Mean
      | (Variable Frequency)
  Mean (Variable Frequency)2 : spsMeanVariableFrequencyLib/Mean (Variable Frequency)  Finit=sps.Finit  Fmin=sps.Fmin  Vinit=sps.Imag_Init  Ts=Ts
      settings: LibrarySourceBlock=|
      | sps_lib/Sensors and Measurements/Mean
      | (Variable Frequency)
  Rad->Deg. : Gain  Gain=180/pi  SaturateOnIntegerOverflow=on  OutDataTypeStr=Inherit: Same as input  ParamDataTypeStr=Inherit: Same as input
  Real-Imag to Complex : RealImagToComplex
  Selector : Selector  InputPortWidth=2  IndexOptions=Index vector (dialog)  Indices=[1]  OutputSizes=1
  Selector1 : Selector  InputPortWidth=2  IndexOptions=Index vector (dialog)  Indices=[2]  OutputSizes=1
  Mag : Outport  SampleTime=Ts  VectorParamsAs1DForOutWhenUnconnected=off
  Phase : Outport  Port=2  SampleTime=Ts  VectorParamsAs1DForOutWhenUnconnected=off
  wires:
  Rad->Deg./1 -> Phase/1
  Mean (Variable Frequency)1/1 -> Real-Imag to Complex/1
  Freq/1 -> Mean (Variable Frequency)1/1, Mean (Variable Frequency)2/1
  Real-Imag to Complex/1 -> Complex to Magnitude-Angle/1
  Mean (Variable Frequency)2/1 -> Real-Imag to Complex/2
  Complex to Magnitude-Angle/1 -> Mag/1
  Complex to Magnitude-Angle/2 -> Rad->Deg./1
  dq/1 -> Selector/1, Selector1/1  "q"
  Selector/1 -> Mean (Variable Frequency)1/2  "d"
  Selector1/1 -> Mean (Variable Frequency)2/2  "q"

== system dqn_C_PQ_HVsMC/Control _DQn/PLL, Measurements and Transformation1/PLL (3ph)/Model/Variable Frequency Mean value/Model ==
  Freq : Inport  PortDimensions=1
  vq : Inport  Port=2
  Constant : Constant  Value=1/sps.Finit
  Correction subsystem : Subsystem
  Digital Clock : DigitalClock  SampleTime=Ts
  Discrete Variable Time Delay : spsDiscreteVariableTimeDelayLib/Discrete Variable Time Delay  MaxDelay=1/sps.Fmin+Ts  InitialValue=0  Ts=Ts  DFT=on
  Gain : Gain  Gain=Ts  SaturateOnIntegerOverflow=on  OutDataTypeStr=Inherit: Same as input  ParamDataTypeStr=Inherit: Same as input
  Integ4 : DiscreteIntegrator  IntegratorMethod=Integration: Trapezoidal  SampleTime=Ts  ICPrevOutput=DiscIntNeverNeededParam  ICPrevScaledInput=DiscIntNeverNeededParam
  Number of samples per cycle : Fcn  Expr=1/u[1]/Ts
  Product : Product  InputSameDT=on  SaturateOnIntegerOverflow=on  OutDataTypeStr=Inherit: Same as first input
  Relational Operator : RelationalOperator  OutDataTypeStr=boolean  SampleTime=Ts  InputSameDT=off
  Rounding Function : Rounding  Operator=ceil
  Sum5 : Sum  InputSameDT=on  SaturateOnIntegerOverflow=on  OutDataTypeStr=Inherit: Same as first input
  Sum7 : Sum  Inputs=-+  InputSameDT=on  SaturateOnIntegerOverflow=on  OutDataTypeStr=Inherit: Same as first input
  Switch : Switch  Threshold=0.5  SaturateOnIntegerOverflow=off
  To avoid division by zero : Saturate  UpperLimit=1e6  LowerLimit=eps
  Unit Delay1 : UnitDelay  InitialCondition=sps.Vinit  SampleTime=Ts  HasFrameUpgradeWarning=on
  Mean : Outport
  wires:
  Correction subsystem/1(Out) -> Sum5/2
  To avoid division by zero/1 -> Number of samples per cycle/1  "Freq"
  Switch/1 -> Mean/1, Unit Delay1/1
  Sum5/1 -> Switch/1
  Number of samples per cycle/1 -> Correction subsystem/1(N), Rounding Function/1
  Rounding Function/1 -> Correction subsystem/2(F), Gain/1
  Gain/1 -> Discrete Variable Time Delay/2  "Delay"
  Freq/1 -> To avoid division by zero/1, Product/2
  Integ4/1 -> Sum7/2, Discrete Variable Time Delay/1
  Sum7/1 -> Product/1
  Discrete Variable Time Delay/1 -> Sum7/1
  Product/1 -> Sum5/1  "Mean value"
  vq/1 -> Correction subsystem/3(In), Integ4/1
  Digital Clock/1 -> Relational Operator/1
  Unit Delay1/1 -> Switch/3
  Relational Operator/1 -> Switch/2
  Constant/1 -> Relational Operator/2

== system dqn_C_PQ_HVsMC/Control _DQn/PLL, Measurements and Transformation1/PLL (3ph)2/Model/Automatic Gain Control/Positive-Sequence (PLL-Driven) ==
  Freq : Inport  SampleTime=Ts
  dq : Inport  Port=2  SampleTime=Ts
  Complex to Magnitude-Angle : ComplexToMagnitudeAngle
  Mean (Variable Frequency)1 : spsMeanVariableFrequencyLib/Mean (Variable Frequency)  Finit=sps.Finit  Fmin=sps.Fmin  Vinit=sps.Real_Init  Ts=Ts
      settings: LibrarySourceBlock=|
      | sps_lib/Sensors and Measurements/Mean
      | (Variable Frequency)
  Mean (Variable Frequency)2 : spsMeanVariableFrequencyLib/Mean (Variable Frequency)  Finit=sps.Finit  Fmin=sps.Fmin  Vinit=sps.Imag_Init  Ts=Ts
      settings: LibrarySourceBlock=|
      | sps_lib/Sensors and Measurements/Mean
      | (Variable Frequency)
  Rad->Deg. : Gain  Gain=180/pi  SaturateOnIntegerOverflow=on  OutDataTypeStr=Inherit: Same as input  ParamDataTypeStr=Inherit: Same as input
  Real-Imag to Complex : RealImagToComplex
  Selector : Selector  InputPortWidth=2  IndexOptions=Index vector (dialog)  Indices=[1]  OutputSizes=1
  Selector1 : Selector  InputPortWidth=2  IndexOptions=Index vector (dialog)  Indices=[2]  OutputSizes=1
  Mag : Outport  SampleTime=Ts  VectorParamsAs1DForOutWhenUnconnected=off
  Phase : Outport  Port=2  SampleTime=Ts  VectorParamsAs1DForOutWhenUnconnected=off
  wires:
  Rad->Deg./1 -> Phase/1
  Mean (Variable Frequency)1/1 -> Real-Imag to Complex/1
  Freq/1 -> Mean (Variable Frequency)1/1, Mean (Variable Frequency)2/1
  Real-Imag to Complex/1 -> Complex to Magnitude-Angle/1
  Mean (Variable Frequency)2/1 -> Real-Imag to Complex/2
  Complex to Magnitude-Angle/1 -> Mag/1
  Complex to Magnitude-Angle/2 -> Rad->Deg./1
  dq/1 -> Selector/1, Selector1/1  "q"
  Selector/1 -> Mean (Variable Frequency)1/2  "d"
  Selector1/1 -> Mean (Variable Frequency)2/2  "q"

== system dqn_C_PQ_HVsMC/Control _DQn/PLL, Measurements and Transformation1/PLL (3ph)2/Model/Variable Frequency Mean value/Model ==
  Freq : Inport  PortDimensions=1
  vq : Inport  Port=2
  Constant : Constant  Value=1/sps.Finit
  Correction subsystem : Subsystem
  Digital Clock : DigitalClock  SampleTime=Ts
  Discrete Variable Time Delay : spsDiscreteVariableTimeDelayLib/Discrete Variable Time Delay  MaxDelay=1/sps.Fmin+Ts  InitialValue=0  Ts=Ts  DFT=on
  Gain : Gain  Gain=Ts  SaturateOnIntegerOverflow=on  OutDataTypeStr=Inherit: Same as input  ParamDataTypeStr=Inherit: Same as input
  Integ4 : DiscreteIntegrator  IntegratorMethod=Integration: Trapezoidal  SampleTime=Ts  ICPrevOutput=DiscIntNeverNeededParam  ICPrevScaledInput=DiscIntNeverNeededParam
  Number of samples per cycle : Fcn  Expr=1/u[1]/Ts
  Product : Product  InputSameDT=on  SaturateOnIntegerOverflow=on  OutDataTypeStr=Inherit: Same as first input
  Relational Operator : RelationalOperator  OutDataTypeStr=boolean  SampleTime=Ts  InputSameDT=off
  Rounding Function : Rounding  Operator=ceil
  Sum5 : Sum  InputSameDT=on  SaturateOnIntegerOverflow=on  OutDataTypeStr=Inherit: Same as first input
  Sum7 : Sum  Inputs=-+  InputSameDT=on  SaturateOnIntegerOverflow=on  OutDataTypeStr=Inherit: Same as first input
  Switch : Switch  Threshold=0.5  SaturateOnIntegerOverflow=off
  To avoid division by zero : Saturate  UpperLimit=1e6  LowerLimit=eps
  Unit Delay1 : UnitDelay  InitialCondition=sps.Vinit  SampleTime=Ts  HasFrameUpgradeWarning=on
  Mean : Outport
  wires:
  Correction subsystem/1(Out) -> Sum5/2
  To avoid division by zero/1 -> Number of samples per cycle/1  "Freq"
  Switch/1 -> Mean/1, Unit Delay1/1
  Sum5/1 -> Switch/1
  Number of samples per cycle/1 -> Correction subsystem/1(N), Rounding Function/1
  Rounding Function/1 -> Correction subsystem/2(F), Gain/1
  Gain/1 -> Discrete Variable Time Delay/2  "Delay"
  Freq/1 -> To avoid division by zero/1, Product/2
  Integ4/1 -> Sum7/2, Discrete Variable Time Delay/1
  Sum7/1 -> Product/1
  Discrete Variable Time Delay/1 -> Sum7/1
  Product/1 -> Sum5/1  "Mean value"
  vq/1 -> Correction subsystem/3(In), Integ4/1
  Digital Clock/1 -> Relational Operator/1
  Unit Delay1/1 -> Switch/3
  Relational Operator/1 -> Switch/2
  Constant/1 -> Relational Operator/2
